simulink model "model"  (R2016a)
(part 2 of 2)

  bus92 : powerlib/Measurements/Load Flow Bus  LConnTagsString=a  Phases=single  Connectors=on one side  ID=bus92  Vbase=220000  Vref=1  Vangle=0  VLF=1  VLFb=1  VLFc=1  angleLF=0  angleLFb=0  angleLFc=0
      settings: AttributesFormatString=|
      | %<ID>
      | %<Vbase>V
      | %<VLF>pu
      | %<angleLF>deg.
      | %<Name>
  bus93 : powerlib/Measurements/Load Flow Bus  LConnTagsString=a  Phases=single  Connectors=on one side  ID=bus93  Vbase=220000  Vref=1  Vangle=0  VLF=1  VLFb=1  VLFc=1  angleLF=0  angleLFb=0  angleLFc=0
      settings: AttributesFormatString=|
      | %<ID>
      | %<Vbase>V
      | %<VLF>pu
      | %<angleLF>deg.
      | %<Name>
  bus94 : powerlib/Measurements/Load Flow Bus  LConnTagsString=a  Phases=single  Connectors=on one side  ID=bus94  Vbase=220000  Vref=1  Vangle=0  VLF=1  VLFb=1  VLFc=1  angleLF=0  angleLFb=0  angleLFc=0
      settings: AttributesFormatString=|
      | %<ID>
      | %<Vbase>V
      | %<VLF>pu
      | %<angleLF>deg.
      | %<Name>
  bus95 : powerlib/Measurements/Load Flow Bus  LConnTagsString=a  Phases=single  Connectors=on one side  ID=bus95  Vbase=220000  Vref=1  Vangle=0  VLF=1  VLFb=1  VLFc=1  angleLF=0  angleLFb=0  angleLFc=0
      settings: AttributesFormatString=|
      | %<ID>
      | %<Vbase>V
      | %<VLF>pu
      | %<angleLF>deg.
      | %<Name>
  bus96 : powerlib/Measurements/Load Flow Bus  LConnTagsString=a  Phases=single  Connectors=on one side  ID=bus96  Vbase=220000  Vref=1  Vangle=0  VLF=1  VLFb=1  VLFc=1  angleLF=0  angleLFb=0  angleLFc=0
      settings: AttributesFormatString=|
      | %<ID>
      | %<Vbase>V
      | %<VLF>pu
      | %<angleLF>deg.
      | %<Name>
  bus97 : powerlib/Measurements/Load Flow Bus  LConnTagsString=a  Phases=single  Connectors=on one side  ID=bus97  Vbase=220000  Vref=1  Vangle=0  VLF=1  VLFb=1  VLFc=1  angleLF=0  angleLFb=0  angleLFc=0
      settings: AttributesFormatString=|
      | %<ID>
      | %<Vbase>V
      | %<VLF>pu
      | %<angleLF>deg.
      | %<Name>
  bus98 : powerlib/Measurements/Load Flow Bus  LConnTagsString=a  Phases=single  Connectors=on one side  ID=bus98  Vbase=220000  Vref=1  Vangle=0  VLF=1  VLFb=1  VLFc=1  angleLF=0  angleLFb=0  angleLFc=0
      settings: AttributesFormatString=|
      | %<ID>
      | %<Vbase>V
      | %<VLF>pu
      | %<angleLF>deg.
      | %<Name>
  bus99 : powerlib/Measurements/Load Flow Bus  LConnTagsString=a  Phases=single  Connectors=on one side  ID=bus99  Vbase=220000  Vref=1  Vangle=0  VLF=1  VLFb=1  VLFc=1  angleLF=0  angleLFb=0  angleLFc=0
      settings: AttributesFormatString=|
      | %<ID>
      | %<Vbase>V
      | %<VLF>pu
      | %<angleLF>deg.
      | %<Name>
  powergui : powerlib/powergui  Priority=1  SimulationMode=Phasor  SolverType=Tustin/Backward Euler (TBE)  SampleTime=50e-6  frequency=50  SPID=off  DisableSnubberDevices=off  DisableRonSwitches=off  DisableVfSwitches=off  SwTol=0  DisplayEquations=off  Interpol=off  ExternalGateDelay=off  methode=off  Ts=10  FunctionMessages=off  echomessages=off  HookPort=off  EnableUseOfTLC=off  x0status=blocks  frequencyindice=50  Pbase=3000e6  ErrMax=0.0001  Iterations=50  UnitsV=V  UnitsW=W  buscounter=0  RestoreLinks=warning  ResistiveCurrentMeasurement=off  Frange=[0:2:500]  Ylog=off  Xlog=on  ShowGrid=off  save=off  variable=ZData  structure=0  ZoomFFT=off  StartTime=0.0  cycles=1  DisplayStyle=1  fundamental=60  FreqAxis=off  MaxFrequency=1000  frequencyindicesteady=1  RmsSteady=1  display=off
  connections:
  _CN_105065132_220000_CN_33041399_220000/LConn1 -- T_105065132_220000_APG_Umspannwerk_Salzburg/LConn1 -- Tauern___Salzburg_CN_105065132_220000_CN_38868243_220000/LConn1
  _CN_105065132_220000_CN_33041399_220000/LConn2 -- T_105065132_220000_APG_Umspannwerk_Salzburg/LConn2 -- Tauern___Salzburg_CN_105065132_220000_CN_38868243_220000/LConn2
  _CN_105065132_220000_CN_33041399_220000/LConn3 -- T_105065132_220000_APG_Umspannwerk_Salzburg/LConn3 -- Tauern___Salzburg_CN_105065132_220000_CN_38868243_220000/LConn3 -- bus1/LConn1
  T_33041399__Salzach/LConn1 -- _CN_105065132_220000_CN_33041399_220000/RConn1
  T_33041399__Salzach/LConn2 -- _CN_105065132_220000_CN_33041399_220000/RConn2
  _CN_105065132_220000_CN_33041399_220000/RConn3 -- T_33041399__Salzach/LConn3 -- bus2/LConn1
  Tauern___Salzburg_CN_105065132_220000_CN_38868243_220000/RConn1 -- T_38868243_380000;220000_Tauern/RConn1 -- Tauern___Weißenbach_CN_38868243_220000_CN_89451551_220000/LConn1 -- L_38868243/LConn1 -- _CN_38868243_220000_CN_38821658_220000/LConn1
  Tauern___Salzburg_CN_105065132_220000_CN_38868243_220000/RConn2 -- T_38868243_380000;220000_Tauern/RConn2 -- Tauern___Weißenbach_CN_38868243_220000_CN_89451551_220000/LConn2 -- L_38868243/LConn2 -- _CN_38868243_220000_CN_38821658_220000/LConn2
  Tauern___Salzburg_CN_105065132_220000_CN_38868243_220000/RConn3 -- T_38868243_380000;220000_Tauern/RConn3 -- Tauern___Weißenbach_CN_38868243_220000_CN_89451551_220000/LConn3 -- L_38868243/LConn3 -- bus3/LConn1 -- _CN_38868243_220000_CN_38821658_220000/LConn3
  _CN_86119428_220000_CN_123588260_220000/LConn1 -- T_86119428_220000_KW_Rosegg/LConn1 -- _CN_86119428_220000_CN_86119456_220000/LConn1 -- _CN_86119428_220000_CN_83831570_220000/LConn1 -- _CN_86119428_220000_CN_162826525_220000/LConn1 -- _CN_86119428_220000_CN_180468540_220000/LConn1
  _CN_86119428_220000_CN_123588260_220000/LConn2 -- T_86119428_220000_KW_Rosegg/LConn2 -- _CN_86119428_220000_CN_86119456_220000/LConn2 -- _CN_86119428_220000_CN_83831570_220000/LConn2 -- _CN_86119428_220000_CN_162826525_220000/LConn2 -- _CN_86119428_220000_CN_180468540_220000/LConn2
  _CN_86119428_220000_CN_123588260_220000/LConn3 -- T_86119428_220000_KW_Rosegg/LConn3 -- _CN_86119428_220000_CN_86119456_220000/LConn3 -- _CN_86119428_220000_CN_83831570_220000/LConn3 -- bus4/LConn1 -- _CN_86119428_220000_CN_162826525_220000/LConn3 -- _CN_86119428_220000_CN_180468540_220000/LConn3
  G_123588260_Kraftwerk_Rosegg_St__Jakob/RConn1 -- _CN_86119428_220000_CN_123588260_220000/RConn1
  G_123588260_Kraftwerk_Rosegg_St__Jakob/RConn2 -- _CN_86119428_220000_CN_123588260_220000/RConn2
  _CN_86119428_220000_CN_123588260_220000/RConn3 -- G_123588260_Kraftwerk_Rosegg_St__Jakob/RConn3 -- bus5/LConn1
  _CN_86119428_220000_CN_162826525_220000/RConn1 -- T_162826525_220000;110000_APG_Umspannwerk_Lienz/RConn1 -- Malta_Hauptstufe___Lienz_CN_162826525_220000_CN_83805040_220000/LConn1 -- L_162826525/LConn1
  _CN_86119428_220000_CN_162826525_220000/RConn2 -- T_162826525_220000;110000_APG_Umspannwerk_Lienz/RConn2 -- Malta_Hauptstufe___Lienz_CN_162826525_220000_CN_83805040_220000/LConn2 -- L_162826525/LConn2
  _CN_86119428_220000_CN_162826525_220000/RConn3 -- T_162826525_220000;110000_APG_Umspannwerk_Lienz/RConn3 -- Malta_Hauptstufe___Lienz_CN_162826525_220000_CN_83805040_220000/LConn3 -- L_162826525/LConn3 -- bus6/LConn1
  T_180468540_220000_Umspannwerk_Greuth/LConn1 -- _CN_86119428_220000_CN_180468540_220000/RConn1
  T_180468540_220000_Umspannwerk_Greuth/LConn2 -- _CN_86119428_220000_CN_180468540_220000/RConn2
  _CN_86119428_220000_CN_180468540_220000/RConn3 -- T_180468540_220000_Umspannwerk_Greuth/LConn3 -- bus7/LConn1
  T_86119456_220000_Freistritz/LConn1 -- _CN_86119428_220000_CN_86119456_220000/RConn1
  T_86119456_220000_Freistritz/LConn2 -- _CN_86119428_220000_CN_86119456_220000/RConn2
  _CN_86119428_220000_CN_86119456_220000/RConn3 -- T_86119456_220000_Freistritz/LConn3 -- bus8/LConn1
  _CN_86119428_220000_CN_83831570_220000/RConn1 -- T_83831570_380000;220000;110000_Umspannwerk_Obersielach/RConn1 -- St__Andrä___Obersielach;Zeltweg___Obersielach_CN_83831570_220000_CN_88684218_220000/LConn1 -- St__Andrä___Obersielach;Zeltweg___Obersielach_CN_83831570_220000_CN_88680218_220000/LConn1 -- St__Andrä___Obersielach;Zeltweg___Obersielach_CN_83831570_220000_CN_88381334_220000/LConn1 -- L_83831570/LConn1
  _CN_86119428_220000_CN_83831570_220000/RConn2 -- T_83831570_380000;220000;110000_Umspannwerk_Obersielach/RConn2 -- St__Andrä___Obersielach;Zeltweg___Obersielach_CN_83831570_220000_CN_88684218_220000/LConn2 -- St__Andrä___Obersielach;Zeltweg___Obersielach_CN_83831570_220000_CN_88680218_220000/LConn2 -- St__Andrä___Obersielach;Zeltweg___Obersielach_CN_83831570_220000_CN_88381334_220000/LConn2 -- L_83831570/LConn2
  _CN_86119428_220000_CN_83831570_220000/RConn3 -- T_83831570_380000;220000;110000_Umspannwerk_Obersielach/RConn3 -- St__Andrä___Obersielach;Zeltweg___Obersielach_CN_83831570_220000_CN_88684218_220000/LConn3 -- St__Andrä___Obersielach;Zeltweg___Obersielach_CN_83831570_220000_CN_88680218_220000/LConn3 -- St__Andrä___Obersielach;Zeltweg___Obersielach_CN_83831570_220000_CN_88381334_220000/LConn3 -- L_83831570/LConn3 -- bus9/LConn1
  _CN_95860758_220000_CN_118091356_220000/LConn1 -- T_95860758__/LConn1 -- _CN_95860758_220000_CN_59531071_220000/LConn1
  _CN_95860758_220000_CN_118091356_220000/LConn2 -- T_95860758__/LConn2 -- _CN_95860758_220000_CN_59531071_220000/LConn2
  _CN_95860758_220000_CN_118091356_220000/LConn3 -- T_95860758__/LConn3 -- _CN_95860758_220000_CN_59531071_220000/LConn3 -- bus10/LConn1
  T_118091356__/LConn1 -- _CN_95860758_220000_CN_118091356_220000/RConn1
  T_118091356__/LConn2 -- _CN_95860758_220000_CN_118091356_220000/RConn2
  _CN_95860758_220000_CN_118091356_220000/RConn3 -- T_118091356__/LConn3 -- bus11/LConn1
  _CN_95860758_220000_CN_59531071_220000/RConn1 -- T_59531071_380000;220000;110000_Umspannwerk_Dürnrohr/RConn1 -- _CN_59531071_220000_CN_24253250_220000/LConn1 -- L_59531071/LConn1
  _CN_95860758_220000_CN_59531071_220000/RConn2 -- T_59531071_380000;220000;110000_Umspannwerk_Dürnrohr/RConn2 -- _CN_59531071_220000_CN_24253250_220000/LConn2 -- L_59531071/LConn2
  _CN_95860758_220000_CN_59531071_220000/RConn3 -- T_59531071_380000;220000;110000_Umspannwerk_Dürnrohr/RConn3 -- _CN_59531071_220000_CN_24253250_220000/LConn3 -- L_59531071/LConn3 -- bus12/LConn1
  Kühtai___Silz_CN_95812231_220000_CN_156083802_220000/LConn1 -- T_95812231_220000;110000_/LConn1 -- _CN_95812231_220000_CN_24768685_220000/LConn1 -- _CN_95812231_220000_CN_95812161_220000/LConn1
  Kühtai___Silz_CN_95812231_220000_CN_156083802_220000/LConn2 -- T_95812231_220000;110000_/LConn2 -- _CN_95812231_220000_CN_24768685_220000/LConn2 -- _CN_95812231_220000_CN_95812161_220000/LConn2
  Kühtai___Silz_CN_95812231_220000_CN_156083802_220000/LConn3 -- T_95812231_220000;110000_/LConn3 -- _CN_95812231_220000_CN_24768685_220000/LConn3 -- bus13/LConn1 -- _CN_95812231_220000_CN_95812161_220000/LConn3
  G_156083802_Kraftwerk_Kühtai/RConn1 -- Kühtai___Silz_CN_95812231_220000_CN_156083802_220000/RConn1
  G_156083802_Kraftwerk_Kühtai/RConn2 -- Kühtai___Silz_CN_95812231_220000_CN_156083802_220000/RConn2
  Kühtai___Silz_CN_95812231_220000_CN_156083802_220000/RConn3 -- G_156083802_Kraftwerk_Kühtai/RConn3 -- bus14/LConn1
  _CN_95812231_220000_CN_95812161_220000/RConn1 -- T_95812161_380000;220000;110000_APG_Umspannwerk_Westtirol/RConn1 -- Westtirol___Zell_am_Ziller_CN_95812161_220000_CN_156973414_220000/LConn1 -- L_95812161/LConn1 -- Prutz___Westtirol_CN_100602290_220000_CN_95812161_220000/LConn1 -- _CN_95812161_220000_CN_101997887_220000/LConn1
  _CN_95812231_220000_CN_95812161_220000/RConn2 -- T_95812161_380000;220000;110000_APG_Umspannwerk_Westtirol/RConn2 -- Westtirol___Zell_am_Ziller_CN_95812161_220000_CN_156973414_220000/LConn2 -- L_95812161/LConn2 -- Prutz___Westtirol_CN_100602290_220000_CN_95812161_220000/LConn2 -- _CN_95812161_220000_CN_101997887_220000/LConn2
  _CN_95812231_220000_CN_95812161_220000/RConn3 -- T_95812161_380000;220000;110000_APG_Umspannwerk_Westtirol/RConn3 -- Westtirol___Zell_am_Ziller_CN_95812161_220000_CN_156973414_220000/LConn3 -- L_95812161/LConn3 -- bus15/LConn1 -- Prutz___Westtirol_CN_100602290_220000_CN_95812161_220000/LConn3 -- _CN_95812161_220000_CN_101997887_220000/LConn3
  _CN_95812231_220000_CN_24768685_220000/RConn1 -- T_24768685_220000;110000_Umspannwerk_Thaur/LConn1 -- Thaur___Strass_CN_24768685_220000_CN_84789829_220000/LConn1
  _CN_95812231_220000_CN_24768685_220000/RConn2 -- T_24768685_220000;110000_Umspannwerk_Thaur/LConn2 -- Thaur___Strass_CN_24768685_220000_CN_84789829_220000/LConn2
  _CN_95812231_220000_CN_24768685_220000/RConn3 -- T_24768685_220000;110000_Umspannwerk_Thaur/LConn3 -- Thaur___Strass_CN_24768685_220000_CN_84789829_220000/LConn3 -- bus16/LConn1
  T_70497801_220000_/LConn1 -- Ybbsfeld___Ybbs_Persenbeug_CN_70497801_220000_CN_30076588_220000/LConn1
  T_70497801_220000_/LConn2 -- Ybbsfeld___Ybbs_Persenbeug_CN_70497801_220000_CN_30076588_220000/LConn2
  Ybbsfeld___Ybbs_Persenbeug_CN_70497801_220000_CN_30076588_220000/LConn3 -- T_70497801_220000_/LConn3 -- bus17/LConn1
  Ybbsfeld___Ybbs_Persenbeug_CN_70497801_220000_CN_30076588_220000/RConn1 -- T_30076588_220000;110000_Umspannwerk_Ybbsfeld/LConn1 -- Ybbsfeld___Bisamberg_CN_30076588_220000_CN_24253250_220000/LConn1 -- _CN_27763479_220000_CN_30076588_220000/LConn1
  Ybbsfeld___Ybbs_Persenbeug_CN_70497801_220000_CN_30076588_220000/RConn2 -- T_30076588_220000;110000_Umspannwerk_Ybbsfeld/LConn2 -- Ybbsfeld___Bisamberg_CN_30076588_220000_CN_24253250_220000/LConn2 -- _CN_27763479_220000_CN_30076588_220000/LConn2
  Ybbsfeld___Ybbs_Persenbeug_CN_70497801_220000_CN_30076588_220000/RConn3 -- T_30076588_220000;110000_Umspannwerk_Ybbsfeld/LConn3 -- Ybbsfeld___Bisamberg_CN_30076588_220000_CN_24253250_220000/LConn3 -- bus18/LConn1 -- _CN_27763479_220000_CN_30076588_220000/LConn3
  T_88684218__Kraftwerk_Zeltweg/LConn1 -- St__Andrä___Obersielach;Zeltweg___Obersielach_CN_83831570_220000_CN_88684218_220000/RConn1
  T_88684218__Kraftwerk_Zeltweg/LConn2 -- St__Andrä___Obersielach;Zeltweg___Obersielach_CN_83831570_220000_CN_88684218_220000/RConn2
  St__Andrä___Obersielach;Zeltweg___Obersielach_CN_83831570_220000_CN_88684218_220000/RConn3 -- T_88684218__Kraftwerk_Zeltweg/LConn3 -- bus19/LConn1
  St__Andrä___Obersielach;Zeltweg___Obersielach_CN_83831570_220000_CN_88680218_220000/RConn1 -- T_88680218_220000;110000_Umspannwerk_Hessenberg/LConn1 -- Hessenberg___Ternitz_CN_88680218_220000_CN_83202471_220000/LConn1 -- Hessenberg___Weißenbach_CN_88680218_220000_CN_89451551_220000/LConn1
  St__Andrä___Obersielach;Zeltweg___Obersielach_CN_83831570_220000_CN_88680218_220000/RConn2 -- T_88680218_220000;110000_Umspannwerk_Hessenberg/LConn2 -- Hessenberg___Ternitz_CN_88680218_220000_CN_83202471_220000/LConn2 -- Hessenberg___Weißenbach_CN_88680218_220000_CN_89451551_220000/LConn2
  St__Andrä___Obersielach;Zeltweg___Obersielach_CN_83831570_220000_CN_88680218_220000/RConn3 -- T_88680218_220000;110000_Umspannwerk_Hessenberg/LConn3 -- Hessenberg___Ternitz_CN_88680218_220000_CN_83202471_220000/LConn3 -- bus20/LConn1 -- Hessenberg___Weißenbach_CN_88680218_220000_CN_89451551_220000/LConn3
  T_88381334_220000_KW_Sankt_Andrä/LConn1 -- St__Andrä___Obersielach;Zeltweg___Obersielach_CN_83831570_220000_CN_88381334_220000/RConn1
  T_88381334_220000_KW_Sankt_Andrä/LConn2 -- St__Andrä___Obersielach;Zeltweg___Obersielach_CN_83831570_220000_CN_88381334_220000/RConn2
  St__Andrä___Obersielach;Zeltweg___Obersielach_CN_83831570_220000_CN_88381334_220000/RConn3 -- T_88381334_220000_KW_Sankt_Andrä/LConn3 -- bus21/LConn1
  T_38821658_380000;220000;110000_Umspannwerk_Kaprun/LConn1 -- _CN_38868243_220000_CN_38821658_220000/RConn1
  T_38821658_380000;220000;110000_Umspannwerk_Kaprun/LConn2 -- _CN_38868243_220000_CN_38821658_220000/RConn2
  _CN_38868243_220000_CN_38821658_220000/RConn3 -- T_38821658_380000;220000;110000_Umspannwerk_Kaprun/LConn3 -- bus22/LConn1
  Tauern___Weißenbach_CN_38868243_220000_CN_89451551_220000/RConn1 -- T_89451551__Umspannwerk_Weißenbach/LConn1 -- Hessenberg___Weißenbach_CN_88680218_220000_CN_89451551_220000/RConn1 -- _CN_27763479_220000_CN_89451551_220000/LConn1
  Tauern___Weißenbach_CN_38868243_220000_CN_89451551_220000/RConn2 -- T_89451551__Umspannwerk_Weißenbach/LConn2 -- Hessenberg___Weißenbach_CN_88680218_220000_CN_89451551_220000/RConn2 -- _CN_27763479_220000_CN_89451551_220000/LConn2
  Tauern___Weißenbach_CN_38868243_220000_CN_89451551_220000/RConn3 -- T_89451551__Umspannwerk_Weißenbach/LConn3 -- Hessenberg___Weißenbach_CN_88680218_220000_CN_89451551_220000/RConn3 -- bus23/LConn1 -- _CN_27763479_220000_CN_89451551_220000/LConn3
  _CN_27763479_220000_CN_89451551_220000/RConn1 -- T_27763479_380000;220000;110000_Umspannwerk_Ernsthofen/RConn1 -- _CN_27763479_220000_CN_30076588_220000/RConn1 -- L_27763479/LConn1 -- _CN_27763479_220000_CN_50650855_220000/LConn1
  _CN_27763479_220000_CN_89451551_220000/RConn2 -- T_27763479_380000;220000;110000_Umspannwerk_Ernsthofen/RConn2 -- _CN_27763479_220000_CN_30076588_220000/RConn2 -- L_27763479/LConn2 -- _CN_27763479_220000_CN_50650855_220000/LConn2
  _CN_27763479_220000_CN_89451551_220000/RConn3 -- T_27763479_380000;220000;110000_Umspannwerk_Ernsthofen/RConn3 -- _CN_27763479_220000_CN_30076588_220000/RConn3 -- L_27763479/LConn3 -- bus24/LConn1 -- _CN_27763479_220000_CN_50650855_220000/LConn3
  T_50650855__Umspannwerk_Sattledt/LConn1 -- _CN_27763479_220000_CN_50650855_220000/RConn1
  T_50650855__Umspannwerk_Sattledt/LConn2 -- _CN_27763479_220000_CN_50650855_220000/RConn2
  _CN_27763479_220000_CN_50650855_220000/RConn3 -- T_50650855__Umspannwerk_Sattledt/LConn3 -- bus25/LConn1
  T_23899163_220000;110000_Umspannwerk_Kirchbichl/LConn1 -- Strass___Kirchbichl_CN_23899163_220000_CN_84789829_220000/LConn1
  T_23899163_220000;110000_Umspannwerk_Kirchbichl/LConn2 -- Strass___Kirchbichl_CN_23899163_220000_CN_84789829_220000/LConn2
  Strass___Kirchbichl_CN_23899163_220000_CN_84789829_220000/LConn3 -- T_23899163_220000;110000_Umspannwerk_Kirchbichl/LConn3 -- bus26/LConn1
  Strass___Kirchbichl_CN_23899163_220000_CN_84789829_220000/RConn1 -- T_84789829_220000_Schaltwerk_Strass/LConn1 -- Thaur___Strass_CN_24768685_220000_CN_84789829_220000/RConn1 -- Strass___Zell_CN_84789829_220000_CN_156973414_220000/LConn1
  Strass___Kirchbichl_CN_23899163_220000_CN_84789829_220000/RConn2 -- T_84789829_220000_Schaltwerk_Strass/LConn2 -- Thaur___Strass_CN_24768685_220000_CN_84789829_220000/RConn2 -- Strass___Zell_CN_84789829_220000_CN_156973414_220000/LConn2
  Strass___Kirchbichl_CN_23899163_220000_CN_84789829_220000/RConn3 -- T_84789829_220000_Schaltwerk_Strass/LConn3 -- Thaur___Strass_CN_24768685_220000_CN_84789829_220000/RConn3 -- Strass___Zell_CN_84789829_220000_CN_156973414_220000/LConn3 -- bus27/LConn1
  Hessenberg___Ternitz_CN_88680218_220000_CN_83202471_220000/RConn1 -- T_83202471_220000;110000_Umspannwerk_Ternitz/LConn1 -- Ternitz___Wien_Südost_CN_83202471_220000_CN_27795895_220000/LConn1
  Hessenberg___Ternitz_CN_88680218_220000_CN_83202471_220000/RConn2 -- T_83202471_220000;110000_Umspannwerk_Ternitz/LConn2 -- Ternitz___Wien_Südost_CN_83202471_220000_CN_27795895_220000/LConn2
  Hessenberg___Ternitz_CN_88680218_220000_CN_83202471_220000/RConn3 -- T_83202471_220000;110000_Umspannwerk_Ternitz/LConn3 -- Ternitz___Wien_Südost_CN_83202471_220000_CN_27795895_220000/LConn3 -- bus28/LConn1
  T_33631653_220000_Umspannwerk_Greifenstein/LConn1 -- Greifenstein___Bisamberg_CN_33631653_220000_CN_24253250_220000/LConn1
  T_33631653_220000_Umspannwerk_Greifenstein/LConn2 -- Greifenstein___Bisamberg_CN_33631653_220000_CN_24253250_220000/LConn2
  Greifenstein___Bisamberg_CN_33631653_220000_CN_24253250_220000/LConn3 -- T_33631653_220000_Umspannwerk_Greifenstein/LConn3 -- bus29/LConn1
  Greifenstein___Bisamberg_CN_33631653_220000_CN_24253250_220000/RConn1 -- T_24253250_380000;220000;110000_Umspannwerk_Bisamberg/RConn1 -- Ybbsfeld___Bisamberg_CN_30076588_220000_CN_24253250_220000/RConn1 -- _CN_27795895_220000_CN_24253250_220000/LConn1 -- _CN_59531071_220000_CN_24253250_220000/RConn1 -- L_24253250/LConn1
  Greifenstein___Bisamberg_CN_33631653_220000_CN_24253250_220000/RConn2 -- T_24253250_380000;220000;110000_Umspannwerk_Bisamberg/RConn2 -- Ybbsfeld___Bisamberg_CN_30076588_220000_CN_24253250_220000/RConn2 -- _CN_27795895_220000_CN_24253250_220000/LConn2 -- _CN_59531071_220000_CN_24253250_220000/RConn2 -- L_24253250/LConn2
  Greifenstein___Bisamberg_CN_33631653_220000_CN_24253250_220000/RConn3 -- T_24253250_380000;220000;110000_Umspannwerk_Bisamberg/RConn3 -- Ybbsfeld___Bisamberg_CN_30076588_220000_CN_24253250_220000/RConn3 -- _CN_27795895_220000_CN_24253250_220000/LConn3 -- _CN_59531071_220000_CN_24253250_220000/RConn3 -- L_24253250/LConn3 -- bus30/LConn1
  Ternitz___Wien_Südost_CN_83202471_220000_CN_27795895_220000/RConn1 -- T_27795895_380000;220000;110000_Umspannwerk_Wien_Südost/RConn1 -- _CN_27795895_220000_CN_82201785_220000/LConn1 -- L_27795895/LConn1 -- _CN_27795895_220000_CN_24253250_220000/RConn1
  Ternitz___Wien_Südost_CN_83202471_220000_CN_27795895_220000/RConn2 -- T_27795895_380000;220000;110000_Umspannwerk_Wien_Südost/RConn2 -- _CN_27795895_220000_CN_82201785_220000/LConn2 -- L_27795895/LConn2 -- _CN_27795895_220000_CN_24253250_220000/RConn2
  Ternitz___Wien_Südost_CN_83202471_220000_CN_27795895_220000/RConn3 -- T_27795895_380000;220000;110000_Umspannwerk_Wien_Südost/RConn3 -- _CN_27795895_220000_CN_82201785_220000/LConn3 -- L_27795895/LConn3 -- bus31/LConn1 -- _CN_27795895_220000_CN_24253250_220000/RConn3
  T_92873353_220000_/LConn1 -- _CN_92873353_220000_CN_81540198_220000/LConn1
  T_92873353_220000_/LConn2 -- _CN_92873353_220000_CN_81540198_220000/LConn2
  _CN_92873353_220000_CN_81540198_220000/LConn3 -- T_92873353_220000_/LConn3 -- bus32/LConn1
  _CN_92873353_220000_CN_81540198_220000/RConn1 -- T_81540198__Umspannwerk_St__Peter/RConn1 -- _CN_50729129_220000_CN_81540198_220000/LConn1 -- L_81540198/LConn1
  _CN_92873353_220000_CN_81540198_220000/RConn2 -- T_81540198__Umspannwerk_St__Peter/RConn2 -- _CN_50729129_220000_CN_81540198_220000/LConn2 -- L_81540198/LConn2
  _CN_92873353_220000_CN_81540198_220000/RConn3 -- T_81540198__Umspannwerk_St__Peter/RConn3 -- _CN_50729129_220000_CN_81540198_220000/LConn3 -- L_81540198/LConn3 -- bus33/LConn1
  _CN_50729129_220000_CN_210191809_220000/LConn1 -- T_50729129_220000_Jochenstein/LConn1 -- _CN_50729129_220000_CN_81540198_220000/RConn1
  _CN_50729129_220000_CN_210191809_220000/LConn2 -- T_50729129_220000_Jochenstein/LConn2 -- _CN_50729129_220000_CN_81540198_220000/RConn2
  _CN_50729129_220000_CN_210191809_220000/LConn3 -- T_50729129_220000_Jochenstein/LConn3 -- _CN_50729129_220000_CN_81540198_220000/RConn3 -- bus34/LConn1
  T_210191809_220000_Freiluftschaltanlage_KW_Schärding_Neuhaus/LConn1 -- _CN_50729129_220000_CN_210191809_220000/RConn1
  T_210191809_220000_Freiluftschaltanlage_KW_Schärding_Neuhaus/LConn2 -- _CN_50729129_220000_CN_210191809_220000/RConn2
  _CN_50729129_220000_CN_210191809_220000/RConn3 -- T_210191809_220000_Freiluftschaltanlage_KW_Schärding_Neuhaus/LConn3 -- bus35/LConn1
  Malta_Hauptstufe___Lienz_CN_162826525_220000_CN_83805040_220000/RConn1 -- T_83805040_220000;110000_KW_Malta_Hauptstufe/LConn1 -- _CN_83805040_220000_CN_83805041_220000/LConn1
  Malta_Hauptstufe___Lienz_CN_162826525_220000_CN_83805040_220000/RConn2 -- T_83805040_220000;110000_KW_Malta_Hauptstufe/LConn2 -- _CN_83805040_220000_CN_83805041_220000/LConn2
  Malta_Hauptstufe___Lienz_CN_162826525_220000_CN_83805040_220000/RConn3 -- T_83805040_220000;110000_KW_Malta_Hauptstufe/LConn3 -- _CN_83805040_220000_CN_83805041_220000/LConn3 -- bus36/LConn1
  T_100602290_220000;110000_Kraftwerk_Prutz/LConn1 -- Prutz___Westtirol_CN_100602290_220000_CN_95812161_220000/RConn1
  T_100602290_220000;110000_Kraftwerk_Prutz/LConn2 -- Prutz___Westtirol_CN_100602290_220000_CN_95812161_220000/RConn2
  Prutz___Westtirol_CN_100602290_220000_CN_95812161_220000/RConn3 -- T_100602290_220000;110000_Kraftwerk_Prutz/LConn3 -- bus37/LConn1
  Rodund_II___Bürs_CN_219909161_220000_CN_101997887_220000/LConn1 -- T_219909161__Umspannwerk_Rodund_II/LConn1 -- Rodund_II___Bürs_CN_219909161_220000_CN_219909160_220000/LConn1
  Rodund_II___Bürs_CN_219909161_220000_CN_101997887_220000/LConn2 -- T_219909161__Umspannwerk_Rodund_II/LConn2 -- Rodund_II___Bürs_CN_219909161_220000_CN_219909160_220000/LConn2
  Rodund_II___Bürs_CN_219909161_220000_CN_101997887_220000/LConn3 -- T_219909161__Umspannwerk_Rodund_II/LConn3 -- Rodund_II___Bürs_CN_219909161_220000_CN_219909160_220000/LConn3 -- bus38/LConn1
  Rodund_II___Bürs_CN_219909161_220000_CN_101997887_220000/RConn1 -- T_101997887_380000;220000_Umspannwerk_Bürs/RConn1 -- _CN_95812161_220000_CN_101997887_220000/RConn1 -- Meiningen___Werben_blau_CN_61108302_220000_CN_101997887_220000/LConn1 -- _CN_83529203_220000_CN_101997887_220000/LConn1 -- L_101997887/LConn1
  Rodund_II___Bürs_CN_219909161_220000_CN_101997887_220000/RConn2 -- T_101997887_380000;220000_Umspannwerk_Bürs/RConn2 -- _CN_95812161_220000_CN_101997887_220000/RConn2 -- Meiningen___Werben_blau_CN_61108302_220000_CN_101997887_220000/LConn2 -- _CN_83529203_220000_CN_101997887_220000/LConn2 -- L_101997887/LConn2
  Rodund_II___Bürs_CN_219909161_220000_CN_101997887_220000/RConn3 -- T_101997887_380000;220000_Umspannwerk_Bürs/RConn3 -- _CN_95812161_220000_CN_101997887_220000/RConn3 -- Meiningen___Werben_blau_CN_61108302_220000_CN_101997887_220000/LConn3 -- _CN_83529203_220000_CN_101997887_220000/LConn3 -- L_101997887/LConn3 -- bus39/LConn1
  T_219909160__/LConn1 -- Rodund_II___Bürs_CN_219909161_220000_CN_219909160_220000/RConn1
  T_219909160__/LConn2 -- Rodund_II___Bürs_CN_219909161_220000_CN_219909160_220000/RConn2
  Rodund_II___Bürs_CN_219909161_220000_CN_219909160_220000/RConn3 -- T_219909160__/LConn3 -- bus40/LConn1
  T_82201785_220000;110000_Umspannwerk_Neusiedl/LConn1 -- _CN_27795895_220000_CN_82201785_220000/RConn1
  T_82201785_220000;110000_Umspannwerk_Neusiedl/LConn2 -- _CN_27795895_220000_CN_82201785_220000/RConn2
  _CN_27795895_220000_CN_82201785_220000/RConn3 -- T_82201785_220000;110000_Umspannwerk_Neusiedl/LConn3 -- bus41/LConn1
  Westtirol___Zell_am_Ziller_CN_95812161_220000_CN_156973414_220000/RConn1 -- T_156973414_380000;220000;110000_Umspannwerk_Zell_am_Ziller/RConn1 -- Strass___Zell_CN_84789829_220000_CN_156973414_220000/RConn1 -- Mayrhofen___Zell_CN_156973414_220000_CN_28596524_220000/LConn1 -- L_156973414/LConn1
  Westtirol___Zell_am_Ziller_CN_95812161_220000_CN_156973414_220000/RConn2 -- T_156973414_380000;220000;110000_Umspannwerk_Zell_am_Ziller/RConn2 -- Strass___Zell_CN_84789829_220000_CN_156973414_220000/RConn2 -- Mayrhofen___Zell_CN_156973414_220000_CN_28596524_220000/LConn2 -- L_156973414/LConn2
  Westtirol___Zell_am_Ziller_CN_95812161_220000_CN_156973414_220000/RConn3 -- T_156973414_380000;220000;110000_Umspannwerk_Zell_am_Ziller/RConn3 -- Strass___Zell_CN_84789829_220000_CN_156973414_220000/RConn3 -- Mayrhofen___Zell_CN_156973414_220000_CN_28596524_220000/LConn3 -- L_156973414/LConn3 -- bus42/LConn1
  Meiningen___Werben_blau_CN_61108302_220000_CN_83529203_220000/LConn1 -- T_61108302_380000;220000_Umspannwerk_Meiningen/LConn1 -- Meiningen___Werben_blau_CN_61108302_220000_CN_101997887_220000/RConn1
  Meiningen___Werben_blau_CN_61108302_220000_CN_83529203_220000/LConn2 -- T_61108302_380000;220000_Umspannwerk_Meiningen/LConn2 -- Meiningen___Werben_blau_CN_61108302_220000_CN_101997887_220000/RConn2
  Meiningen___Werben_blau_CN_61108302_220000_CN_83529203_220000/LConn3 -- T_61108302_380000;220000_Umspannwerk_Meiningen/LConn3 -- Meiningen___Werben_blau_CN_61108302_220000_CN_101997887_220000/RConn3 -- bus43/LConn1
  Meiningen___Werben_blau_CN_61108302_220000_CN_83529203_220000/RConn1 -- T_83529203_380000;220000_Umspannwerk_Werben___Dornbirn/LConn1 -- _CN_83529203_220000_CN_101997887_220000/RConn1
  Meiningen___Werben_blau_CN_61108302_220000_CN_83529203_220000/RConn2 -- T_83529203_380000;220000_Umspannwerk_Werben___Dornbirn/LConn2 -- _CN_83529203_220000_CN_101997887_220000/RConn2
  Meiningen___Werben_blau_CN_61108302_220000_CN_83529203_220000/RConn3 -- T_83529203_380000;220000_Umspannwerk_Werben___Dornbirn/LConn3 -- _CN_83529203_220000_CN_101997887_220000/RConn3 -- bus44/LConn1
  Mayrhofen___Zell_CN_156973414_220000_CN_28596524_220000/RConn1 -- T_28596524_220000_/LConn1 -- _CN_28596524_220000_CN_62238576_220000/LConn1
  Mayrhofen___Zell_CN_156973414_220000_CN_28596524_220000/RConn2 -- T_28596524_220000_/LConn2 -- _CN_28596524_220000_CN_62238576_220000/LConn2
  Mayrhofen___Zell_CN_156973414_220000_CN_28596524_220000/RConn3 -- T_28596524_220000_/LConn3 -- _CN_28596524_220000_CN_62238576_220000/LConn3 -- bus45/LConn1
  G_83805041_Kraftstation_Rottau/RConn1 -- _CN_83805040_220000_CN_83805041_220000/RConn1
  G_83805041_Kraftstation_Rottau/RConn2 -- _CN_83805040_220000_CN_83805041_220000/RConn2
  _CN_83805040_220000_CN_83805041_220000/RConn3 -- G_83805041_Kraftstation_Rottau/RConn3 -- bus46/LConn1
  G_62238576_Kraftwerk_Häusling/RConn1 -- _CN_28596524_220000_CN_62238576_220000/RConn1
  G_62238576_Kraftwerk_Häusling/RConn2 -- _CN_28596524_220000_CN_62238576_220000/RConn2
  _CN_28596524_220000_CN_62238576_220000/RConn3 -- G_62238576_Kraftwerk_Häusling/RConn3 -- bus47/LConn1
  _CN_107248400_380000_CN_171066516_380000/LConn1 -- T_107248400_380000;110000_Umspannwerk_Sarasdorf/LConn1 -- _CN_107248400_380000_CN_27795895_380000/LConn1 -- _CN_107248400_380000_CN_24253250_380000/LConn1 -- _CN_107248400_380000_CN_59531071_380000/LConn1
  _CN_107248400_380000_CN_171066516_380000/LConn2 -- T_107248400_380000;110000_Umspannwerk_Sarasdorf/LConn2 -- _CN_107248400_380000_CN_27795895_380000/LConn2 -- _CN_107248400_380000_CN_24253250_380000/LConn2 -- _CN_107248400_380000_CN_59531071_380000/LConn2
  _CN_107248400_380000_CN_171066516_380000/LConn3 -- T_107248400_380000;110000_Umspannwerk_Sarasdorf/LConn3 -- _CN_107248400_380000_CN_27795895_380000/LConn3 -- bus48/LConn1 -- _CN_107248400_380000_CN_24253250_380000/LConn3 -- _CN_107248400_380000_CN_59531071_380000/LConn3
  T_171066516_380000;110000_Umspannwerk_Zurndorf/LConn1 -- _CN_107248400_380000_CN_171066516_380000/RConn1
  T_171066516_380000;110000_Umspannwerk_Zurndorf/LConn2 -- _CN_107248400_380000_CN_171066516_380000/RConn2
  _CN_107248400_380000_CN_171066516_380000/RConn3 -- T_171066516_380000;110000_Umspannwerk_Zurndorf/LConn3 -- bus49/LConn1
  _CN_107248400_380000_CN_24253250_380000/RConn1 -- T_24253250_380000;220000;110000_Umspannwerk_Bisamberg/LConn1 -- Bisamberg___Wien_Nord_2_CN_119489306_380000_CN_24253250_380000/LConn1
  _CN_107248400_380000_CN_24253250_380000/RConn2 -- T_24253250_380000;220000;110000_Umspannwerk_Bisamberg/LConn2 -- Bisamberg___Wien_Nord_2_CN_119489306_380000_CN_24253250_380000/LConn2
  _CN_107248400_380000_CN_24253250_380000/RConn3 -- T_24253250_380000;220000;110000_Umspannwerk_Bisamberg/LConn3 -- Bisamberg___Wien_Nord_2_CN_119489306_380000_CN_24253250_380000/LConn3 -- bus50/LConn1
  _CN_107248400_380000_CN_59531071_380000/RConn1 -- T_59531071_380000;220000;110000_Umspannwerk_Dürnrohr/LConn1 -- Ernsthofen___Etzersdorf_CN_30042006_380000_CN_59531071_380000/LConn1 -- _CN_122592181_380000_CN_59531071_380000/LConn1
  _CN_107248400_380000_CN_59531071_380000/RConn2 -- T_59531071_380000;220000;110000_Umspannwerk_Dürnrohr/LConn2 -- Ernsthofen___Etzersdorf_CN_30042006_380000_CN_59531071_380000/LConn2 -- _CN_122592181_380000_CN_59531071_380000/LConn2
  _CN_107248400_380000_CN_59531071_380000/RConn3 -- T_59531071_380000;220000;110000_Umspannwerk_Dürnrohr/LConn3 -- Ernsthofen___Etzersdorf_CN_30042006_380000_CN_59531071_380000/LConn3 -- _CN_122592181_380000_CN_59531071_380000/LConn3 -- bus51/LConn1
  _CN_107248400_380000_CN_27795895_380000/RConn1 -- T_27795895_380000;220000;110000_Umspannwerk_Wien_Südost/LConn1 -- _CN_134565164_380000_CN_27795895_380000/LConn1
  _CN_107248400_380000_CN_27795895_380000/RConn2 -- T_27795895_380000;220000;110000_Umspannwerk_Wien_Südost/LConn2 -- _CN_134565164_380000_CN_27795895_380000/LConn2
  _CN_107248400_380000_CN_27795895_380000/RConn3 -- T_27795895_380000;220000;110000_Umspannwerk_Wien_Südost/LConn3 -- _CN_134565164_380000_CN_27795895_380000/LConn3 -- bus52/LConn1
  T_83831570_380000;220000;110000_Umspannwerk_Obersielach/LConn1 -- Obersielach___Kainachtal_CN_83831570_380000_CN_83740194_380000/LConn1
  T_83831570_380000;220000;110000_Umspannwerk_Obersielach/LConn2 -- Obersielach___Kainachtal_CN_83831570_380000_CN_83740194_380000/LConn2
  Obersielach___Kainachtal_CN_83831570_380000_CN_83740194_380000/LConn3 -- T_83831570_380000;220000;110000_Umspannwerk_Obersielach/LConn3 -- bus53/LConn1
  Obersielach___Kainachtal_CN_83831570_380000_CN_83740194_380000/RConn1 -- T_83740194_380000;110000_Umspannwerk_Kainachtal_Zwaring/LConn1 -- _CN_81684898_380000_CN_83740194_380000/LConn1
  Obersielach___Kainachtal_CN_83831570_380000_CN_83740194_380000/RConn2 -- T_83740194_380000;110000_Umspannwerk_Kainachtal_Zwaring/LConn2 -- _CN_81684898_380000_CN_83740194_380000/LConn2
  Obersielach___Kainachtal_CN_83831570_380000_CN_83740194_380000/RConn3 -- T_83740194_380000;110000_Umspannwerk_Kainachtal_Zwaring/LConn3 -- _CN_81684898_380000_CN_83740194_380000/LConn3 -- bus54/LConn1
  _CN_38868243_380000_CN_318616912_380000/LConn1 -- T_38868243_380000;220000_Tauern/LConn1 -- _CN_38868243_380000_CN_156973414_380000/LConn1 -- _CN_38868243_380000_CN_162826525_380000/LConn1
  _CN_38868243_380000_CN_318616912_380000/LConn2 -- T_38868243_380000;220000_Tauern/LConn2 -- _CN_38868243_380000_CN_156973414_380000/LConn2 -- _CN_38868243_380000_CN_162826525_380000/LConn2
  _CN_38868243_380000_CN_318616912_380000/LConn3 -- T_38868243_380000;220000_Tauern/LConn3 -- _CN_38868243_380000_CN_156973414_380000/LConn3 -- _CN_38868243_380000_CN_162826525_380000/LConn3 -- bus55/LConn1
  T_318616912__Umspannwerk_Schwarzenbach/LConn1 -- _CN_38868243_380000_CN_318616912_380000/RConn1
  T_318616912__Umspannwerk_Schwarzenbach/LConn2 -- _CN_38868243_380000_CN_318616912_380000/RConn2
  _CN_38868243_380000_CN_318616912_380000/RConn3 -- T_318616912__Umspannwerk_Schwarzenbach/LConn3 -- bus56/LConn1
  T_156973414_380000;220000;110000_Umspannwerk_Zell_am_Ziller/LConn1 -- _CN_38868243_380000_CN_156973414_380000/RConn1
  T_156973414_380000;220000;110000_Umspannwerk_Zell_am_Ziller/LConn2 -- _CN_38868243_380000_CN_156973414_380000/RConn2
  _CN_38868243_380000_CN_156973414_380000/RConn3 -- T_156973414_380000;220000;110000_Umspannwerk_Zell_am_Ziller/LConn3 -- bus57/LConn1
  T_162826525_220000;110000_APG_Umspannwerk_Lienz/LConn1 -- _CN_38868243_380000_CN_162826525_380000/RConn1
  T_162826525_220000;110000_APG_Umspannwerk_Lienz/LConn2 -- _CN_38868243_380000_CN_162826525_380000/RConn2
  _CN_38868243_380000_CN_162826525_380000/RConn3 -- T_162826525_220000;110000_APG_Umspannwerk_Lienz/LConn3 -- bus58/LConn1
  _CN_30042006_380000_CN_27797285_380000/LConn1 -- T_30042006_380000_Schaltwerk_Etzersdorf/LConn1 -- Ernsthofen___Etzersdorf_CN_30042006_380000_CN_59531071_380000/RConn1 -- _CN_30042006_380000_CN_47001881_380000/LConn1 -- Ernsthofen___Etzersdorf_CN_30042006_380000_CN_235546807_380000/LConn1
  _CN_30042006_380000_CN_27797285_380000/LConn2 -- T_30042006_380000_Schaltwerk_Etzersdorf/LConn2 -- Ernsthofen___Etzersdorf_CN_30042006_380000_CN_59531071_380000/RConn2 -- _CN_30042006_380000_CN_47001881_380000/LConn2 -- Ernsthofen___Etzersdorf_CN_30042006_380000_CN_235546807_380000/LConn2
  _CN_30042006_380000_CN_27797285_380000/LConn3 -- T_30042006_380000_Schaltwerk_Etzersdorf/LConn3 -- Ernsthofen___Etzersdorf_CN_30042006_380000_CN_59531071_380000/RConn3 -- bus59/LConn1 -- _CN_30042006_380000_CN_47001881_380000/LConn3 -- Ernsthofen___Etzersdorf_CN_30042006_380000_CN_235546807_380000/LConn3
  T_27797285_380000;110000_Umspannwerk_Pottenbrunn/LConn1 -- _CN_30042006_380000_CN_27797285_380000/RConn1
  T_27797285_380000;110000_Umspannwerk_Pottenbrunn/LConn2 -- _CN_30042006_380000_CN_27797285_380000/RConn2
  _CN_30042006_380000_CN_27797285_380000/RConn3 -- T_27797285_380000;110000_Umspannwerk_Pottenbrunn/LConn3 -- bus60/LConn1
  T_47001881_380000;110000_Umspannwerk_Theiß/LConn1 -- _CN_30042006_380000_CN_47001881_380000/RConn1
  T_47001881_380000;110000_Umspannwerk_Theiß/LConn2 -- _CN_30042006_380000_CN_47001881_380000/RConn2
  _CN_30042006_380000_CN_47001881_380000/RConn3 -- T_47001881_380000;110000_Umspannwerk_Theiß/LConn3 -- bus61/LConn1
  Ernsthofen___Etzersdorf_CN_30042006_380000_CN_235546807_380000/RConn1 -- T_235546807_380000_Schaltwerk_Kronstorf/LConn1 -- St__Peter___Ernsthofen_CN_235546807_380000_CN_81540198_380000/LConn1 -- _CN_27763479_380000_CN_235546807_380000/LConn1
  Ernsthofen___Etzersdorf_CN_30042006_380000_CN_235546807_380000/RConn2 -- T_235546807_380000_Schaltwerk_Kronstorf/LConn2 -- St__Peter___Ernsthofen_CN_235546807_380000_CN_81540198_380000/LConn2 -- _CN_27763479_380000_CN_235546807_380000/LConn2
  Ernsthofen___Etzersdorf_CN_30042006_380000_CN_235546807_380000/RConn3 -- T_235546807_380000_Schaltwerk_Kronstorf/LConn3 -- St__Peter___Ernsthofen_CN_235546807_380000_CN_81540198_380000/LConn3 -- bus62/LConn1 -- _CN_27763479_380000_CN_235546807_380000/LConn3
  T_27763479_380000;220000;110000_Umspannwerk_Ernsthofen/LConn1 -- _CN_27763479_380000_CN_235546807_380000/RConn1
  T_27763479_380000;220000;110000_Umspannwerk_Ernsthofen/LConn2 -- _CN_27763479_380000_CN_235546807_380000/RConn2
  _CN_27763479_380000_CN_235546807_380000/RConn3 -- T_27763479_380000;220000;110000_Umspannwerk_Ernsthofen/LConn3 -- bus63/LConn1
  T_119489306_380000_Kabelüberführungsstation_380kV_1GW_Nordeinspeisung/LConn1 -- Bisamberg___Wien_Nord_2_CN_119489306_380000_CN_24253250_380000/RConn1
  T_119489306_380000_Kabelüberführungsstation_380kV_1GW_Nordeinspeisung/LConn2 -- Bisamberg___Wien_Nord_2_CN_119489306_380000_CN_24253250_380000/RConn2
  Bisamberg___Wien_Nord_2_CN_119489306_380000_CN_24253250_380000/RConn3 -- T_119489306_380000_Kabelüberführungsstation_380kV_1GW_Nordeinspeisung/LConn3 -- bus64/LConn1
  _CN_81684898_380000_CN_83742801_380000/LConn1 -- T_81684898_380000;110000_Umspannwerk_Südburgenland_Rotenturm/LConn1 -- _CN_81684898_380000_CN_83740194_380000/RConn1
  _CN_81684898_380000_CN_83742801_380000/LConn2 -- T_81684898_380000;110000_Umspannwerk_Südburgenland_Rotenturm/LConn2 -- _CN_81684898_380000_CN_83740194_380000/RConn2
  _CN_81684898_380000_CN_83742801_380000/LConn3 -- T_81684898_380000;110000_Umspannwerk_Südburgenland_Rotenturm/LConn3 -- _CN_81684898_380000_CN_83740194_380000/RConn3 -- bus65/LConn1
  T_83742801_380000;110000_Umspannwerk_Oststeiermark_Wünschendorf/LConn1 -- _CN_81684898_380000_CN_83742801_380000/RConn1
  T_83742801_380000;110000_Umspannwerk_Oststeiermark_Wünschendorf/LConn2 -- _CN_81684898_380000_CN_83742801_380000/RConn2
  _CN_81684898_380000_CN_83742801_380000/RConn3 -- T_83742801_380000;110000_Umspannwerk_Oststeiermark_Wünschendorf/LConn3 -- bus66/LConn1
  _CN_134565164_380000_CN_27795895_380000/RConn1 -- T_134565164_380000_Kabelüberführungsstation_Pfarrgasse/LConn1 -- _CN_134565164_380000_CN_118060597_380000/LConn1
  _CN_134565164_380000_CN_27795895_380000/RConn2 -- T_134565164_380000_Kabelüberführungsstation_Pfarrgasse/LConn2 -- _CN_134565164_380000_CN_118060597_380000/LConn2
  _CN_134565164_380000_CN_27795895_380000/RConn3 -- T_134565164_380000_Kabelüberführungsstation_Pfarrgasse/LConn3 -- _CN_134565164_380000_CN_118060597_380000/LConn3 -- bus67/LConn1
  T_118060597_380000;110000_Umspannwerk_Süd/LConn1 -- _CN_134565164_380000_CN_118060597_380000/RConn1
  T_118060597_380000;110000_Umspannwerk_Süd/LConn2 -- _CN_134565164_380000_CN_118060597_380000/RConn2
  _CN_134565164_380000_CN_118060597_380000/RConn3 -- T_118060597_380000;110000_Umspannwerk_Süd/LConn3 -- bus68/LConn1
  T_122592181_380000_Umspannwerk_Dürnrohr/LConn1 -- _CN_122592181_380000_CN_59531071_380000/RConn1
  T_122592181_380000_Umspannwerk_Dürnrohr/LConn2 -- _CN_122592181_380000_CN_59531071_380000/RConn2
  _CN_122592181_380000_CN_59531071_380000/RConn3 -- T_122592181_380000_Umspannwerk_Dürnrohr/LConn3 -- bus69/LConn1
  T_95812161_380000;220000;110000_APG_Umspannwerk_Westtirol/LConn1 -- _CN_95812161_380000_CN_101997887_380000/LConn1
  T_95812161_380000;220000;110000_APG_Umspannwerk_Westtirol/LConn2 -- _CN_95812161_380000_CN_101997887_380000/LConn2
  _CN_95812161_380000_CN_101997887_380000/LConn3 -- T_95812161_380000;220000;110000_APG_Umspannwerk_Westtirol/LConn3 -- bus70/LConn1
  T_101997887_380000;220000_Umspannwerk_Bürs/LConn1 -- _CN_95812161_380000_CN_101997887_380000/RConn1
  T_101997887_380000;220000_Umspannwerk_Bürs/LConn2 -- _CN_95812161_380000_CN_101997887_380000/RConn2
  _CN_95812161_380000_CN_101997887_380000/RConn3 -- T_101997887_380000;220000_Umspannwerk_Bürs/LConn3 -- bus71/LConn1
  T_81540198__Umspannwerk_St__Peter/LConn1 -- St__Peter___Ernsthofen_CN_235546807_380000_CN_81540198_380000/RConn1
  T_81540198__Umspannwerk_St__Peter/LConn2 -- St__Peter___Ernsthofen_CN_235546807_380000_CN_81540198_380000/RConn2
  St__Peter___Ernsthofen_CN_235546807_380000_CN_81540198_380000/RConn3 -- T_81540198__Umspannwerk_St__Peter/LConn3 -- bus72/LConn1
  T_105065132_220000_APG_Umspannwerk_Salzburg/RConn1 -- L_105065132/LConn1
  T_105065132_220000_APG_Umspannwerk_Salzburg/RConn2 -- L_105065132/LConn2
  L_105065132/LConn3 -- T_105065132_220000_APG_Umspannwerk_Salzburg/RConn3 -- bus73/LConn1
  T_33041399__Salzach/RConn1 -- L_33041399/LConn1
  T_33041399__Salzach/RConn2 -- L_33041399/LConn2
  L_33041399/LConn3 -- T_33041399__Salzach/RConn3 -- bus74/LConn1
  T_86119428_220000_KW_Rosegg/RConn1 -- L_86119428/LConn1
  T_86119428_220000_KW_Rosegg/RConn2 -- L_86119428/LConn2
  L_86119428/LConn3 -- T_86119428_220000_KW_Rosegg/RConn3 -- bus75/LConn1
  T_180468540_220000_Umspannwerk_Greuth/RConn1 -- L_180468540/LConn1
  T_180468540_220000_Umspannwerk_Greuth/RConn2 -- L_180468540/LConn2
  L_180468540/LConn3 -- T_180468540_220000_Umspannwerk_Greuth/RConn3 -- bus76/LConn1
  T_86119456_220000_Freistritz/RConn1 -- L_86119456/LConn1
  T_86119456_220000_Freistritz/RConn2 -- L_86119456/LConn2
  L_86119456/LConn3 -- T_86119456_220000_Freistritz/RConn3 -- bus77/LConn1
  T_95860758__/RConn1 -- L_95860758/LConn1
  T_95860758__/RConn2 -- L_95860758/LConn2
  L_95860758/LConn3 -- T_95860758__/RConn3 -- bus78/LConn1
  T_118091356__/RConn1 -- L_118091356/LConn1
  T_118091356__/RConn2 -- L_118091356/LConn2
  L_118091356/LConn3 -- T_118091356__/RConn3 -- bus79/LConn1
  T_95812231_220000;110000_/RConn1 -- L_95812231/LConn1
  T_95812231_220000;110000_/RConn2 -- L_95812231/LConn2
  L_95812231/LConn3 -- T_95812231_220000;110000_/RConn3 -- bus80/LConn1
  T_24768685_220000;110000_Umspannwerk_Thaur/RConn1 -- L_24768685/LConn1
  T_24768685_220000;110000_Umspannwerk_Thaur/RConn2 -- L_24768685/LConn2
  L_24768685/LConn3 -- T_24768685_220000;110000_Umspannwerk_Thaur/RConn3 -- bus81/LConn1
  T_70497801_220000_/RConn1 -- L_70497801/LConn1
  T_70497801_220000_/RConn2 -- L_70497801/LConn2
  L_70497801/LConn3 -- T_70497801_220000_/RConn3 -- bus82/LConn1
  T_30076588_220000;110000_Umspannwerk_Ybbsfeld/RConn1 -- L_30076588/LConn1
  T_30076588_220000;110000_Umspannwerk_Ybbsfeld/RConn2 -- L_30076588/LConn2
  L_30076588/LConn3 -- T_30076588_220000;110000_Umspannwerk_Ybbsfeld/RConn3 -- bus83/LConn1
  T_88684218__Kraftwerk_Zeltweg/RConn1 -- L_88684218/LConn1
  T_88684218__Kraftwerk_Zeltweg/RConn2 -- L_88684218/LConn2
  L_88684218/LConn3 -- T_88684218__Kraftwerk_Zeltweg/RConn3 -- bus84/LConn1
  T_88680218_220000;110000_Umspannwerk_Hessenberg/RConn1 -- L_88680218/LConn1
  T_88680218_220000;110000_Umspannwerk_Hessenberg/RConn2 -- L_88680218/LConn2
  L_88680218/LConn3 -- T_88680218_220000;110000_Umspannwerk_Hessenberg/RConn3 -- bus85/LConn1
  T_88381334_220000_KW_Sankt_Andrä/RConn1 -- L_88381334/LConn1
  T_88381334_220000_KW_Sankt_Andrä/RConn2 -- L_88381334/LConn2
  L_88381334/LConn3 -- T_88381334_220000_KW_Sankt_Andrä/RConn3 -- bus86/LConn1
  T_38821658_380000;220000;110000_Umspannwerk_Kaprun/RConn1 -- L_38821658/LConn1
  T_38821658_380000;220000;110000_Umspannwerk_Kaprun/RConn2 -- L_38821658/LConn2
  L_38821658/LConn3 -- T_38821658_380000;220000;110000_Umspannwerk_Kaprun/RConn3 -- bus87/LConn1
  T_89451551__Umspannwerk_Weißenbach/RConn1 -- L_89451551/LConn1
  T_89451551__Umspannwerk_Weißenbach/RConn2 -- L_89451551/LConn2
  L_89451551/LConn3 -- T_89451551__Umspannwerk_Weißenbach/RConn3 -- bus88/LConn1
  T_50650855__Umspannwerk_Sattledt/RConn1 -- L_50650855/LConn1
  T_50650855__Umspannwerk_Sattledt/RConn2 -- L_50650855/LConn2
  L_50650855/LConn3 -- T_50650855__Umspannwerk_Sattledt/RConn3 -- bus89/LConn1
  T_23899163_220000;110000_Umspannwerk_Kirchbichl/RConn1 -- L_23899163/LConn1
  T_23899163_220000;110000_Umspannwerk_Kirchbichl/RConn2 -- L_23899163/LConn2
  L_23899163/LConn3 -- T_23899163_220000;110000_Umspannwerk_Kirchbichl/RConn3 -- bus90/LConn1
  T_84789829_220000_Schaltwerk_Strass/RConn1 -- L_84789829/LConn1
  T_84789829_220000_Schaltwerk_Strass/RConn2 -- L_84789829/LConn2
  L_84789829/LConn3 -- T_84789829_220000_Schaltwerk_Strass/RConn3 -- bus91/LConn1
  T_83202471_220000;110000_Umspannwerk_Ternitz/RConn1 -- L_83202471/LConn1
  T_83202471_220000;110000_Umspannwerk_Ternitz/RConn2 -- L_83202471/LConn2
  L_83202471/LConn3 -- T_83202471_220000;110000_Umspannwerk_Ternitz/RConn3 -- bus92/LConn1
  T_33631653_220000_Umspannwerk_Greifenstein/RConn1 -- L_33631653/LConn1
  T_33631653_220000_Umspannwerk_Greifenstein/RConn2 -- L_33631653/LConn2
  L_33631653/LConn3 -- T_33631653_220000_Umspannwerk_Greifenstein/RConn3 -- bus93/LConn1
  T_92873353_220000_/RConn1 -- L_92873353/LConn1
  T_92873353_220000_/RConn2 -- L_92873353/LConn2
  L_92873353/LConn3 -- T_92873353_220000_/RConn3 -- bus94/LConn1
  T_50729129_220000_Jochenstein/RConn1 -- L_50729129/LConn1
  T_50729129_220000_Jochenstein/RConn2 -- L_50729129/LConn2
  L_50729129/LConn3 -- T_50729129_220000_Jochenstein/RConn3 -- bus95/LConn1
  T_210191809_220000_Freiluftschaltanlage_KW_Schärding_Neuhaus/RConn1 -- L_210191809/LConn1
  T_210191809_220000_Freiluftschaltanlage_KW_Schärding_Neuhaus/RConn2 -- L_210191809/LConn2
  L_210191809/LConn3 -- T_210191809_220000_Freiluftschaltanlage_KW_Schärding_Neuhaus/RConn3 -- bus96/LConn1
  T_83805040_220000;110000_KW_Malta_Hauptstufe/RConn1 -- L_83805040/LConn1
  T_83805040_220000;110000_KW_Malta_Hauptstufe/RConn2 -- L_83805040/LConn2
  L_83805040/LConn3 -- T_83805040_220000;110000_KW_Malta_Hauptstufe/RConn3 -- bus97/LConn1
  T_100602290_220000;110000_Kraftwerk_Prutz/RConn1 -- L_100602290/LConn1
  T_100602290_220000;110000_Kraftwerk_Prutz/RConn2 -- L_100602290/LConn2
  L_100602290/LConn3 -- T_100602290_220000;110000_Kraftwerk_Prutz/RConn3 -- bus98/LConn1
  T_219909161__Umspannwerk_Rodund_II/RConn1 -- L_219909161/LConn1
  T_219909161__Umspannwerk_Rodund_II/RConn2 -- L_219909161/LConn2
  L_219909161/LConn3 -- T_219909161__Umspannwerk_Rodund_II/RConn3 -- bus99/LConn1
  T_219909160__/RConn1 -- L_219909160/LConn1
  T_219909160__/RConn2 -- L_219909160/LConn2
  L_219909160/LConn3 -- T_219909160__/RConn3 -- bus100/LConn1
  T_82201785_220000;110000_Umspannwerk_Neusiedl/RConn1 -- L_82201785/LConn1
  T_82201785_220000;110000_Umspannwerk_Neusiedl/RConn2 -- L_82201785/LConn2
  L_82201785/LConn3 -- T_82201785_220000;110000_Umspannwerk_Neusiedl/RConn3 -- bus101/LConn1
  T_61108302_380000;220000_Umspannwerk_Meiningen/RConn1 -- L_61108302/LConn1
  T_61108302_380000;220000_Umspannwerk_Meiningen/RConn2 -- L_61108302/LConn2
  L_61108302/LConn3 -- T_61108302_380000;220000_Umspannwerk_Meiningen/RConn3 -- bus102/LConn1
  T_83529203_380000;220000_Umspannwerk_Werben___Dornbirn/RConn1 -- L_83529203/LConn1
  T_83529203_380000;220000_Umspannwerk_Werben___Dornbirn/RConn2 -- L_83529203/LConn2
  L_83529203/LConn3 -- T_83529203_380000;220000_Umspannwerk_Werben___Dornbirn/RConn3 -- bus103/LConn1
  T_28596524_220000_/RConn1 -- L_28596524/LConn1
  T_28596524_220000_/RConn2 -- L_28596524/LConn2
  L_28596524/LConn3 -- T_28596524_220000_/RConn3 -- bus104/LConn1
  T_107248400_380000;110000_Umspannwerk_Sarasdorf/RConn1 -- L_107248400/LConn1
  T_107248400_380000;110000_Umspannwerk_Sarasdorf/RConn2 -- L_107248400/LConn2
  L_107248400/LConn3 -- T_107248400_380000;110000_Umspannwerk_Sarasdorf/RConn3 -- bus105/LConn1
  T_171066516_380000;110000_Umspannwerk_Zurndorf/RConn1 -- L_171066516/LConn1
  T_171066516_380000;110000_Umspannwerk_Zurndorf/RConn2 -- L_171066516/LConn2
  L_171066516/LConn3 -- T_171066516_380000;110000_Umspannwerk_Zurndorf/RConn3 -- bus106/LConn1
  T_83740194_380000;110000_Umspannwerk_Kainachtal_Zwaring/RConn1 -- L_83740194/LConn1
  T_83740194_380000;110000_Umspannwerk_Kainachtal_Zwaring/RConn2 -- L_83740194/LConn2
  L_83740194/LConn3 -- T_83740194_380000;110000_Umspannwerk_Kainachtal_Zwaring/RConn3 -- bus107/LConn1
  T_318616912__Umspannwerk_Schwarzenbach/RConn1 -- L_318616912/LConn1
  T_318616912__Umspannwerk_Schwarzenbach/RConn2 -- L_318616912/LConn2
  L_318616912/LConn3 -- T_318616912__Umspannwerk_Schwarzenbach/RConn3 -- bus108/LConn1
  T_30042006_380000_Schaltwerk_Etzersdorf/RConn1 -- L_30042006/LConn1
  T_30042006_380000_Schaltwerk_Etzersdorf/RConn2 -- L_30042006/LConn2
  L_30042006/LConn3 -- T_30042006_380000_Schaltwerk_Etzersdorf/RConn3 -- bus109/LConn1
  T_27797285_380000;110000_Umspannwerk_Pottenbrunn/RConn1 -- L_27797285/LConn1
  T_27797285_380000;110000_Umspannwerk_Pottenbrunn/RConn2 -- L_27797285/LConn2
  L_27797285/LConn3 -- T_27797285_380000;110000_Umspannwerk_Pottenbrunn/RConn3 -- bus110/LConn1
  T_47001881_380000;110000_Umspannwerk_Theiß/RConn1 -- L_47001881/LConn1
  T_47001881_380000;110000_Umspannwerk_Theiß/RConn2 -- L_47001881/LConn2
  L_47001881/LConn3 -- T_47001881_380000;110000_Umspannwerk_Theiß/RConn3 -- bus111/LConn1
  T_235546807_380000_Schaltwerk_Kronstorf/RConn1 -- L_235546807/LConn1
  T_235546807_380000_Schaltwerk_Kronstorf/RConn2 -- L_235546807/LConn2
  L_235546807/LConn3 -- T_235546807_380000_Schaltwerk_Kronstorf/RConn3 -- bus112/LConn1
  T_119489306_380000_Kabelüberführungsstation_380kV_1GW_Nordeinspeisung/RConn1 -- L_119489306/LConn1
  T_119489306_380000_Kabelüberführungsstation_380kV_1GW_Nordeinspeisung/RConn2 -- L_119489306/LConn2
  L_119489306/LConn3 -- T_119489306_380000_Kabelüberführungsstation_380kV_1GW_Nordeinspeisung/RConn3 -- bus113/LConn1
  T_81684898_380000;110000_Umspannwerk_Südburgenland_Rotenturm/RConn1 -- L_81684898/LConn1
  T_81684898_380000;110000_Umspannwerk_Südburgenland_Rotenturm/RConn2 -- L_81684898/LConn2
  L_81684898/LConn3 -- T_81684898_380000;110000_Umspannwerk_Südburgenland_Rotenturm/RConn3 -- bus114/LConn1
  T_83742801_380000;110000_Umspannwerk_Oststeiermark_Wünschendorf/RConn1 -- L_83742801/LConn1
  T_83742801_380000;110000_Umspannwerk_Oststeiermark_Wünschendorf/RConn2 -- L_83742801/LConn2
  L_83742801/LConn3 -- T_83742801_380000;110000_Umspannwerk_Oststeiermark_Wünschendorf/RConn3 -- bus115/LConn1
  T_134565164_380000_Kabelüberführungsstation_Pfarrgasse/RConn1 -- L_134565164/LConn1
  T_134565164_380000_Kabelüberführungsstation_Pfarrgasse/RConn2 -- L_134565164/LConn2
  L_134565164/LConn3 -- T_134565164_380000_Kabelüberführungsstation_Pfarrgasse/RConn3 -- bus116/LConn1
  T_118060597_380000;110000_Umspannwerk_Süd/RConn1 -- L_118060597/LConn1
  T_118060597_380000;110000_Umspannwerk_Süd/RConn2 -- L_118060597/LConn2
  L_118060597/LConn3 -- T_118060597_380000;110000_Umspannwerk_Süd/RConn3 -- bus117/LConn1
  T_122592181_380000_Umspannwerk_Dürnrohr/RConn1 -- L_122592181/LConn1
  T_122592181_380000_Umspannwerk_Dürnrohr/RConn2 -- L_122592181/LConn2
  L_122592181/LConn3 -- T_122592181_380000_Umspannwerk_Dürnrohr/RConn3 -- bus118/LConn1
